simulink model "VAB_Linear_PolePlacement"  (R2019b)
settings: Solver=FixedStepAuto  StartTime=0.0  StopTime=t_end  FixedStep=Ts  RelTol=1e-3
values from neighbouring files (symbols this model uses):
  K = [-0.00227126037234 -0.0278341382787 -28.1396904229 -7.70218039791]    [K.mat]
undefined symbols (not defined in the file or in its folder): A_real, B_real, C_real, control_on, sigbuilder_block, x_0
settings Model: Creator=miche  LastModifiedBy=miche

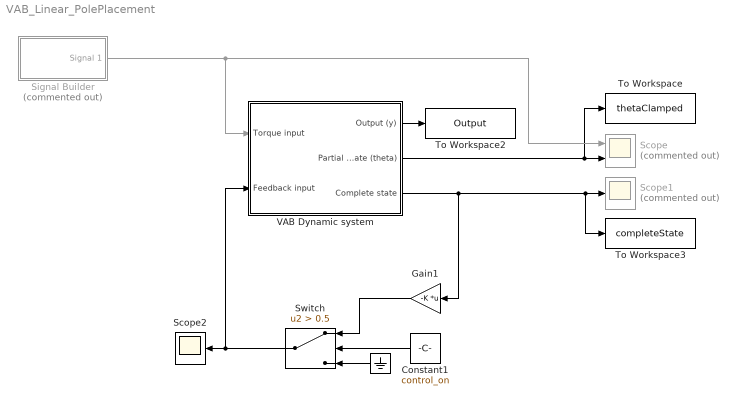
== system VAB_Linear_PolePlacement ==
  " " : Ground
  Constant1 : Constant  Value=control_on
  Gain1 : Gain  Gain=-K  Multiplication=Matrix(K*u)
  Scope : Scope  Commented=on  NumInputPorts=2
  Scope1 : Scope  Commented=on
  Scope2 : Scope
  Signal Builder : Subsystem  Tag=STV Subsys  Commented=on  LoadFcn=sigbuilder_block('load');  StartFcn=sigbuilder_block('start');  StopFcn=sigbuilder_block('stop');  ClipboardFcn=sigbuilder_block('clipboard');  mask(Sigbuilder block){tuvar=[0:10]}
      mask help: Simulink:masks:SigbuilderBlock_MD
      mask init:
      | if ~strcmp(get_param(bdroot(gcbh),'SimulationStatus'),'stopped') tuvar = sigbuilder_block('maskInit'); end
      settings: CopyFcn=sigbuilder_block('copy');  DeleteFcn=sigbuilder_block('delete');  ModelCloseFcn=sigbuilder_block('modelClose');  PreSaveFcn=sigbuilder_block('preSave');  PauseFcn=sigbuilder_block('pause');  ContinueFcn=sigbuilder_block('continue');  NameChangeFcn=sigbuilder_block('namechange');  OpenFcn=sigbuilder_block('open',[6 6 1012.5 506.25 ]);  CloseFcn=sigbuilder_block('close');
      mask Display: plot(0, 0, 100, 100,[2, 2, 32, 32, 2], [68, 8, 8, 68, 68],[32, 2], [38, 38], [32, 19, 2],[53, 60, 44], [32, 17, 17, 2],[16, 16, 31, 31]);txt = getActiveGroup(gcbh);text(2, 100, txt,'verticalAlignment', 'top');
  Switch : Switch  Criteria=u2 > Threshold  Threshold=0.5
  To Workspace : ToWorkspace  VariableName=thetaClamped  SampleTime=-1
  To Workspace2 : ToWorkspace  VariableName=Output  SampleTime=-1
  To Workspace3 : ToWorkspace  VariableName=completeState  SampleTime=-1
  VAB Dynamic system : Subsystem
  wires:
  VAB Dynamic system/3("Complete state ") -> Gain1/1, To Workspace3/1, Scope1/1
  VAB Dynamic system/2(Partial state (theta)) -> To Workspace/1, Scope/2
  VAB Dynamic system/1(Output (y)) -> To Workspace2/1
  Signal Builder/1(Signal 1) -> Scope/1, VAB Dynamic system/1(Torque input)
  Constant1/1 -> Switch/2
  " "/1 -> Switch/3
  Gain1/1 -> Switch/1
  Switch/1 -> Scope2/1, VAB Dynamic system/2(Feedback input)

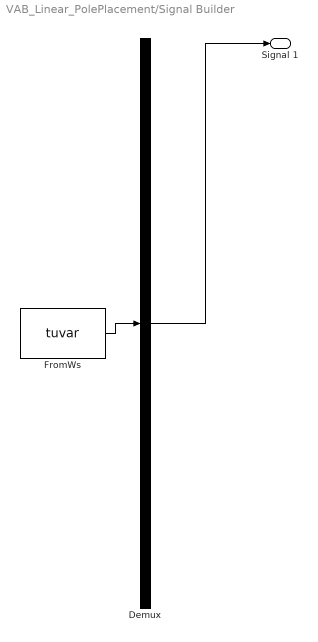
== system VAB_Linear_PolePlacement/Signal Builder ==
  Demux : Demux  Tag=STV Demux  Outputs=1
  FromWs : FromWorkspace  Tag=STV FromWs  VariableName=tuvar  SampleTime=0
      SigBuilderData=|
      | common.afterFinalStr = 'Extrapolate'
      | common.sampleTime = 0
      | dataSet.timeRange = [0 10]
      | dataSet.name = 'Group 1'
      | sbobj.Groups.Name = 'Group 1'
      | sbobj.Groups.Signals.Name = 'Signal 1'
      | sbobj.Groups.Signals.XData = [0 4 4 4.58 4.58 10]
      | sbobj.Groups.Signals.YData = [0 0 0.998 1 0 0]
  Signal 1 : Outport  Tag=STV Outport
  wires:
  Demux/1 -> Signal 1/1
  FromWs/1 -> Demux/1

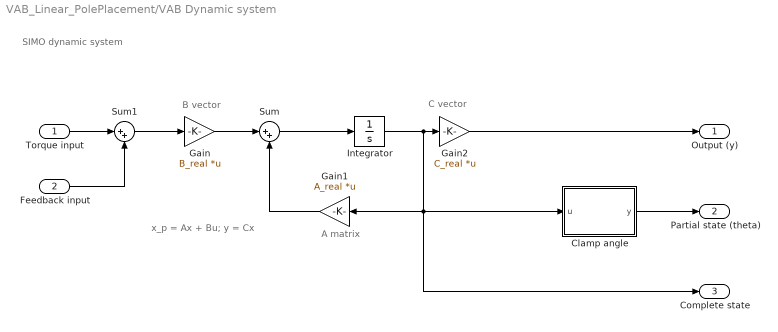
== system VAB_Linear_PolePlacement/VAB Dynamic system ==
  note: C vector
  note: SIMO dynamic system
  note: x_p = Ax + Bu;
      | y = Cx
  note: B vector
  note: A matrix
  Torque input : Inport
  Feedback input : Inport  Port=2
  Clamp angle : MATLAB Function  TreatAsAtomicUnit=on
  Gain : Gain  Gain=B_real  Multiplication=Matrix(K*u)
  Gain1 : Gain  Gain=A_real  Multiplication=Matrix(K*u)
  Gain2 : Gain  Gain=C_real  Multiplication=Matrix(K*u) (u vector)
  Integrator : Integrator  InitialCondition=x_0
  Sum : Sum  Inputs=|++
  Sum1 : Sum  Inputs=|++
  Output (y) : Outport
  Partial state (theta) : Outport  Port=2
  "Complete state " : Outport  Port=3
  wires:
  Gain2/1 -> Output (y)/1
  Gain1/1 -> Sum/2
  Integrator/1 -> Gain2/1, Clamp angle/1(u), "Complete state "/1, Gain1/1
  Gain/1 -> Sum/1
  Sum/1 -> Integrator/1
  Clamp angle/1(y) -> Partial state (theta)/1
  Sum1/1 -> Gain/1
  Feedback input/1 -> Sum1/2
  Torque input/1 -> Sum1/1

== matlab function VAB_Linear_PolePlacement/VAB Dynamic system/Clamp angle ==
  data: u input; y output
function y = fcn(u)

if u(3) ~= 0
   u(3) = mod(u(3), 2 * pi); 
end

y = rad2deg(u(3));
